simulink model "robusni_lin_regulacija_nelin_sim"  (R2020a)
settings: Solver=ode5  StartTime=0.0  StopTime=tfin  FixedStep=1e-4  RelTol=1e-3
values from neighbouring files (symbols this model uses):
  disturb_X = 0    [robusni_lin_regulacija_nelin_sim_matlab.m]
  F_lower_limit = 0    [robusni_lin_regulacija_nelin_sim_matlab.m]
  F_upper_limit = 1e-3*Fe    (= 0.00320891060125)    [robusni_lin_regulacija_nelin_sim_matlab.m]
  Fe = 3.20891060125344    (= 3.20891060125)    [robusni_lin_regulacija_nelin_sim_matlab.m]
  K1 = 0.03    [robusni_lin_regulacija_nelin_sim_matlab.m]
  K2 = 0.5    [robusni_lin_regulacija_nelin_sim_matlab.m]
  Kc1 = 1/abs(freqresp((1+1/Ti1/s)*G_design,w1_design))    [robusni_lin_regulacija_nelin_sim_matlab.m]
  mi_max = 1    [robusni_lin_regulacija_nelin_sim_matlab.m]
  S_step1 = delta    (= 0.0138373075366)    [robusni_lin_regulacija_nelin_sim_matlab.m]
  S_step2 = delta    (= 0.0138373075366)    [robusni_lin_regulacija_nelin_sim_matlab.m]
  S_time_step1 = 20    [robusni_lin_regulacija_nelin_sim_matlab.m]
  S_time_step2 = 50    [robusni_lin_regulacija_nelin_sim_matlab.m]
  Se = 0.218662692463450    (= 0.218662692463)    [robusni_lin_regulacija_nelin_sim_matlab.m]
  SF = 10    [robusni_lin_regulacija_nelin_sim_matlab.m]
  std_noise = 0    [robusni_lin_regulacija_nelin_sim_matlab.m]
  V = 4    [robusni_lin_regulacija_nelin_sim_matlab.m]
  x10 = Xe    (= 4.89066865377)    [robusni_lin_regulacija_nelin_sim_matlab.m]
  x20 = Se    (= 0.218662692463)    [robusni_lin_regulacija_nelin_sim_matlab.m]
  Y = Ynom    (= 0.5)    [robusni_lin_regulacija_nelin_sim_matlab.m]
  Y1 = Y - 0.2*Y    (= 0.4)    [robusni_lin_regulacija_nelin_sim_matlab.m]
  Y2 = Y - 0.1*Y    (= 0.45)    [robusni_lin_regulacija_nelin_sim_matlab.m]
  Y3 = Y + 0.1*Y    (= 0.55)    [robusni_lin_regulacija_nelin_sim_matlab.m]
  Y4 = Y + 0.2*Y    (= 0.6)    [robusni_lin_regulacija_nelin_sim_matlab.m]
undefined symbols (not defined in the file or in its folder): magnitude
libraries: cstblocks x10
settings Model: Creator=anaMceranic  LastModifiedBy=anaMceranic
settings DataIOCC: ReturnWorkspaceOutputs=off

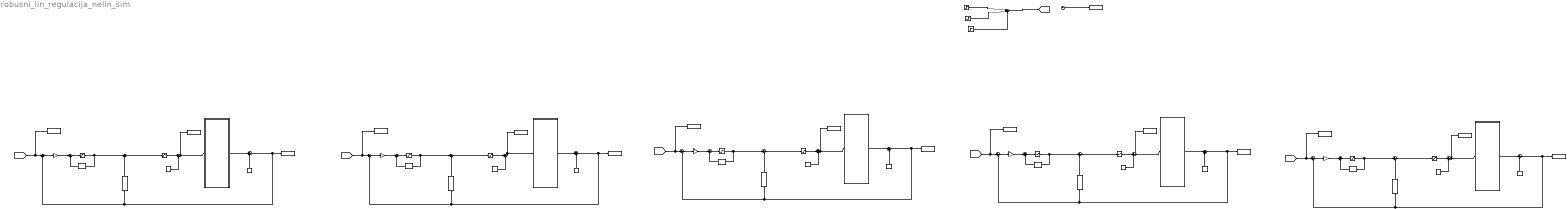
== system robusni_lin_regulacija_nelin_sim ==
  note: 1.2 Y
  note: 1.1 Y
  note: 0.9Y
  note: 0.8Y
  note: nominalni
  Clock : Clock
  Constant{1..5} (5 alike) : Constant  Value=Fe
  Gain{,1..4} (5 alike) : Gain  Gain=Kc1
  LTI System{,2,4,6,8} (5 alike) : cstblocks/LTI System  sys=KPI_aw  IC=[]
  LTI System{1,3,5,7,9} (5 alike) : cstblocks/LTI System  sys=Kfb  IC=[]
  Random Number{,1..4} (5 alike) : RandomNumber  Variance=std_noise  SampleTime=0.1
  Saturation{1..10} (10 alike) : Saturate  UpperLimit=F_upper_limit  LowerLimit=F_lower_limit
  Step2 : Step  Time=0  Before=Se  After=Se  SampleTime=0
  Step3 : Step  Time=S_time_step1  After=S_step1  SampleTime=0
  Step4 : Step  Time=S_time_step2  After=-S_step2  SampleTime=0
  Subsystem1 : Subsystem
  Subsystem2 : Subsystem
  Subsystem3 : Subsystem
  Subsystem4 : Subsystem
  Subsystem5 : Subsystem
  Sum{1..2,4,6,8,11..13,16..18,21..23,26} (15 alike) : Sum  Inputs=|++
  Sum{3,5,9..10,14..15,19..20,24..25} (10 alike) : Sum  Inputs=|+-
  Sum7 : Sum  Inputs=|+++
  To Workspace1 : ToWorkspace  VariableName=t_out  SampleTime=-1
  To Workspace10 : ToWorkspace  VariableName=S_ref_out2  SampleTime=-1
  To Workspace11 : ToWorkspace  VariableName=S_out3  SampleTime=-1
  To Workspace12 : ToWorkspace  VariableName=F_out3  SampleTime=-1
  To Workspace13 : ToWorkspace  VariableName=S_ref_out3  SampleTime=-1
  To Workspace14 : ToWorkspace  VariableName=S_out4  SampleTime=-1
  To Workspace15 : ToWorkspace  VariableName=F_out4  SampleTime=-1
  To Workspace16 : ToWorkspace  VariableName=S_ref_out4  SampleTime=-1
  To Workspace2 : ToWorkspace  VariableName=S_out1  SampleTime=-1
  To Workspace3 : ToWorkspace  VariableName=F_out1  SampleTime=-1
  To Workspace4 : ToWorkspace  VariableName=S_ref_out1  SampleTime=-1
  To Workspace5 : ToWorkspace  VariableName=S_out2  SampleTime=-1
  To Workspace6 : ToWorkspace  VariableName=S_out  SampleTime=-1
  To Workspace7 : ToWorkspace  VariableName=F_out  SampleTime=-1
  To Workspace8 : ToWorkspace  VariableName=S_ref_out  SampleTime=-1
  To Workspace9 : ToWorkspace  VariableName=F_out2  SampleTime=-1
  wires:
  Clock/1 -> To Workspace1/1
  Sum6/1 -> To Workspace7/1, Subsystem2/1(u)
  Saturation1/1 -> Sum6/1
  Constant1/1 -> Sum6/2
  Sum5/1 -> Gain/1
  Sum7/1 -> [S_refere]
  Step2/1 -> Sum7/1
  [S_refere] -> To Workspace8/1, Sum5/1
  Gain/1 -> Sum1/1
  Sum1/1 -> Saturation2/1
  LTI System/1 -> Sum1/2
  Step3/1 -> Sum7/2
  Step4/1 -> Sum7/3
  Subsystem2/1(y) -> Sum2/1
  Sum2/1 -> Sum5/2, LTI System1/1, To Workspace6/1
  Random Number/1 -> Sum2/2
  Saturation2/1 -> Sum3/1, LTI System/1
  Sum3/1 -> Saturation1/1
  LTI System1/1 -> Sum3/2
  Sum4/1 -> Saturation4/1
  Constant2/1 -> Sum11/2
  Sum11/1 -> To Workspace3/1, Subsystem1/1(u)
  Gain1/1 -> Sum4/1
  Sum9/1 -> Saturation3/1
  Saturation4/1 -> Sum9/1, LTI System2/1
  LTI System2/1 -> Sum4/2
  Saturation3/1 -> Sum11/1
  Sum8/1 -> Sum10/2, LTI System3/1, To Workspace2/1
  Random Number1/1 -> Sum8/2
  [S_refere] -> To Workspace4/1, Sum10/1
  LTI System3/1 -> Sum9/2
  Subsystem1/1(y) -> Sum8/1
  Sum10/1 -> Gain1/1
  Sum12/1 -> Saturation6/1
  Constant3/1 -> Sum16/2
  Sum16/1 -> To Workspace9/1, Subsystem3/1(u)
  Gain2/1 -> Sum12/1
  Sum14/1 -> Saturation5/1
  Saturation6/1 -> Sum14/1, LTI System4/1
  LTI System4/1 -> Sum12/2
  Saturation5/1 -> Sum16/1
  Sum13/1 -> Sum15/2, LTI System5/1, To Workspace5/1
  Random Number2/1 -> Sum13/2
  [S_refere] -> To Workspace10/1, Sum15/1
  LTI System5/1 -> Sum14/2
  Subsystem3/1(y) -> Sum13/1
  Sum15/1 -> Gain2/1
  Sum17/1 -> Saturation8/1
  Constant4/1 -> Sum21/2
  Sum21/1 -> To Workspace12/1, Subsystem4/1(u)
  Gain3/1 -> Sum17/1
  Sum19/1 -> Saturation7/1
  Saturation8/1 -> Sum19/1, LTI System6/1
  LTI System6/1 -> Sum17/2
  Saturation7/1 -> Sum21/1
  Sum18/1 -> Sum20/2, LTI System7/1, To Workspace11/1
  Random Number3/1 -> Sum18/2
  [S_refere] -> To Workspace13/1, Sum20/1
  LTI System7/1 -> Sum19/2
  Subsystem4/1(y) -> Sum18/1
  Sum20/1 -> Gain3/1
  Sum22/1 -> Saturation10/1
  Constant5/1 -> Sum26/2
  Sum26/1 -> To Workspace15/1, Subsystem5/1(u)
  Gain4/1 -> Sum22/1
  Sum24/1 -> Saturation9/1
  Saturation10/1 -> Sum24/1, LTI System8/1
  LTI System8/1 -> Sum22/2
  Saturation9/1 -> Sum26/1
  Sum23/1 -> Sum25/2, LTI System9/1, To Workspace14/1
  Random Number4/1 -> Sum23/2
  [S_refere] -> To Workspace16/1, Sum25/1
  LTI System9/1 -> Sum24/2
  Subsystem5/1(y) -> Sum23/1
  Sum25/1 -> Gain4/1

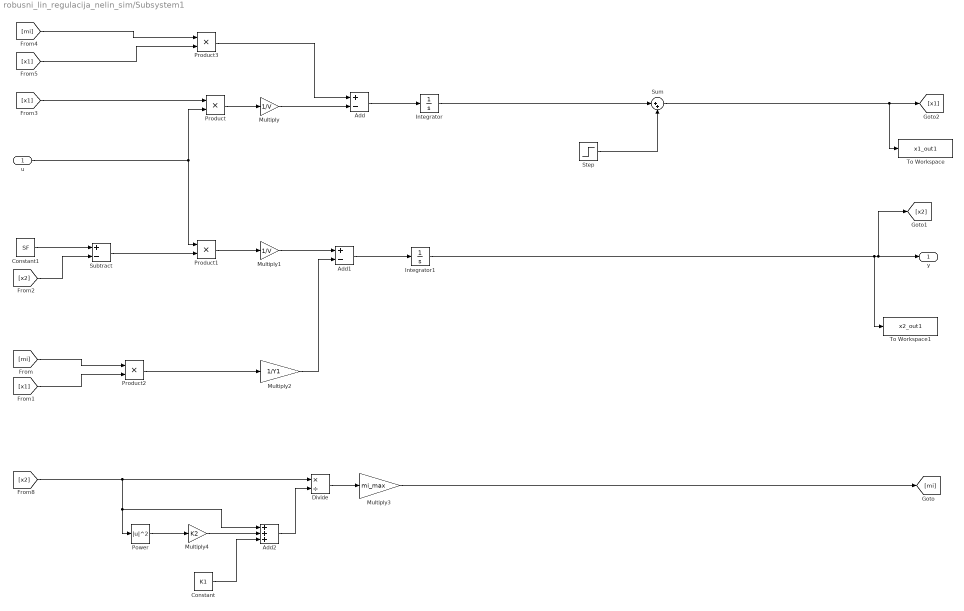
== system robusni_lin_regulacija_nelin_sim/Subsystem1 ==
  u : Inport
  Add : Sum  Inputs=+-
  Add1 : Sum  Inputs=+-
  Add2 : Sum  Inputs=+++
  Constant : Constant  Value=K1
  Constant1 : Constant  Value=SF
  Divide : Product  Inputs=*/
  Integrator : Integrator  InitialCondition=x10
  Integrator1 : Integrator  InitialCondition=x20
  Multiply : Gain  Gain=1/V
  Multiply1 : Gain  Gain=1/V
  Multiply2 : Gain  Gain=1/Y1
  Multiply3 : Gain  Gain=mi_max
  Multiply4 : Gain  Gain=K2
  Power : Math  Operator=magnitude^2  SaturateOnIntegerOverflow=on
  Product{,1..3} (4 alike) : Product
  Step : Step  Time=2  After=disturb_X  SampleTime=0
  Subtract : Sum  Inputs=+-
  Sum : Sum  Inputs=|++
  To Workspace : ToWorkspace  VariableName=x1_out1  SampleTime=-1
  To Workspace1 : ToWorkspace  VariableName=x2_out1  SampleTime=-1
  y : Outport
  wires:
  [x1] -> Product2/2
  Product2/1 -> Multiply2/1
  Multiply/1 -> Add/2
  Add2/1 -> Divide/2
  Constant/1 -> Add2/3
  [x1] -> Product3/2
  Multiply4/1 -> Add2/2
  [mi] -> Product2/1
  Multiply3/1 -> [mi]
  Power/1 -> Multiply4/1
  Constant1/1 -> Subtract/1
  [x2] -> Subtract/2
  Add1/1 -> Integrator1/1
  Multiply2/1 -> Add1/2
  Integrator1/1 -> [x2], y/1, To Workspace1/1
  Divide/1 -> Multiply3/1
  Product3/1 -> Add/1
  u/1 -> Product1/1, Product/2
  [x1] -> Product/1
  Multiply1/1 -> Add1/1
  Product1/1 -> Multiply1/1
  Subtract/1 -> Product1/2
  [x2] -> Divide/1, Add2/1, Power/1
  Add/1 -> Integrator/1
  Product/1 -> Multiply/1
  [mi] -> Product3/1
  Integrator/1 -> Sum/1
  Sum/1 -> To Workspace/1, [x1]
  Step/1 -> Sum/2

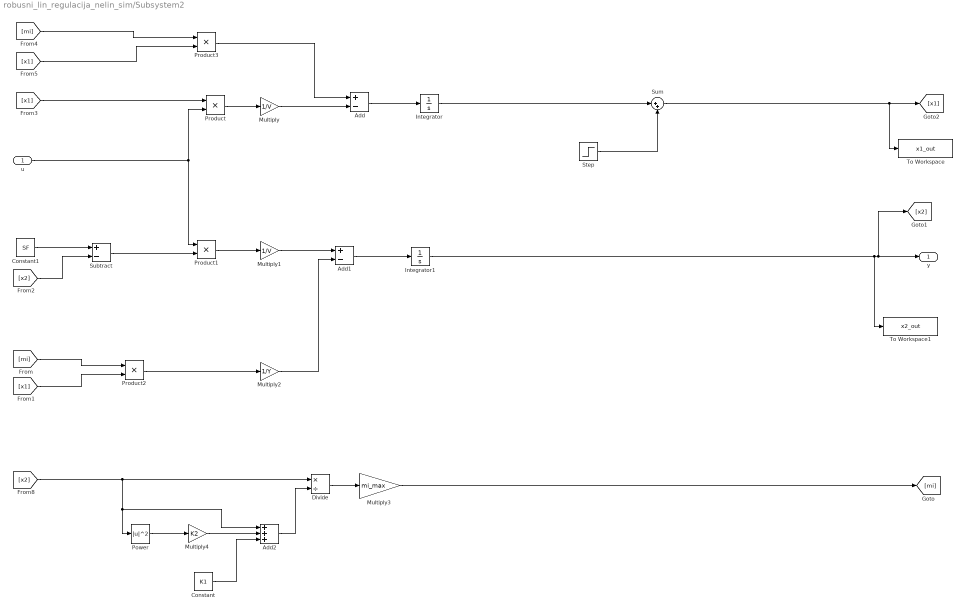
== system robusni_lin_regulacija_nelin_sim/Subsystem2 ==
  u : Inport
  Add : Sum  Inputs=+-
  Add1 : Sum  Inputs=+-
  Add2 : Sum  Inputs=+++
  Constant : Constant  Value=K1
  Constant1 : Constant  Value=SF
  Divide : Product  Inputs=*/
  Integrator : Integrator  InitialCondition=x10
  Integrator1 : Integrator  InitialCondition=x20
  Multiply : Gain  Gain=1/V
  Multiply1 : Gain  Gain=1/V
  Multiply2 : Gain  Gain=1/Y
  Multiply3 : Gain  Gain=mi_max
  Multiply4 : Gain  Gain=K2
  Power : Math  Operator=magnitude^2  SaturateOnIntegerOverflow=on
  Product{,1..3} (4 alike) : Product
  Step : Step  Time=2  After=disturb_X  SampleTime=0
  Subtract : Sum  Inputs=+-
  Sum : Sum  Inputs=|++
  To Workspace : ToWorkspace  VariableName=x1_out  SampleTime=-1
  To Workspace1 : ToWorkspace  VariableName=x2_out  SampleTime=-1
  y : Outport
  wires:
  [x1] -> Product2/2
  Product2/1 -> Multiply2/1
  Multiply/1 -> Add/2
  Add2/1 -> Divide/2
  Constant/1 -> Add2/3
  [x1] -> Product3/2
  Multiply4/1 -> Add2/2
  [mi] -> Product2/1
  Multiply3/1 -> [mi]
  Power/1 -> Multiply4/1
  Constant1/1 -> Subtract/1
  [x2] -> Subtract/2
  Add1/1 -> Integrator1/1
  Multiply2/1 -> Add1/2
  Integrator1/1 -> [x2], y/1, To Workspace1/1
  Divide/1 -> Multiply3/1
  Product3/1 -> Add/1
  u/1 -> Product1/1, Product/2
  [x1] -> Product/1
  Multiply1/1 -> Add1/1
  Product1/1 -> Multiply1/1
  Subtract/1 -> Product1/2
  [x2] -> Divide/1, Add2/1, Power/1
  Add/1 -> Integrator/1
  Product/1 -> Multiply/1
  [mi] -> Product3/1
  Integrator/1 -> Sum/1
  Sum/1 -> To Workspace/1, [x1]
  Step/1 -> Sum/2

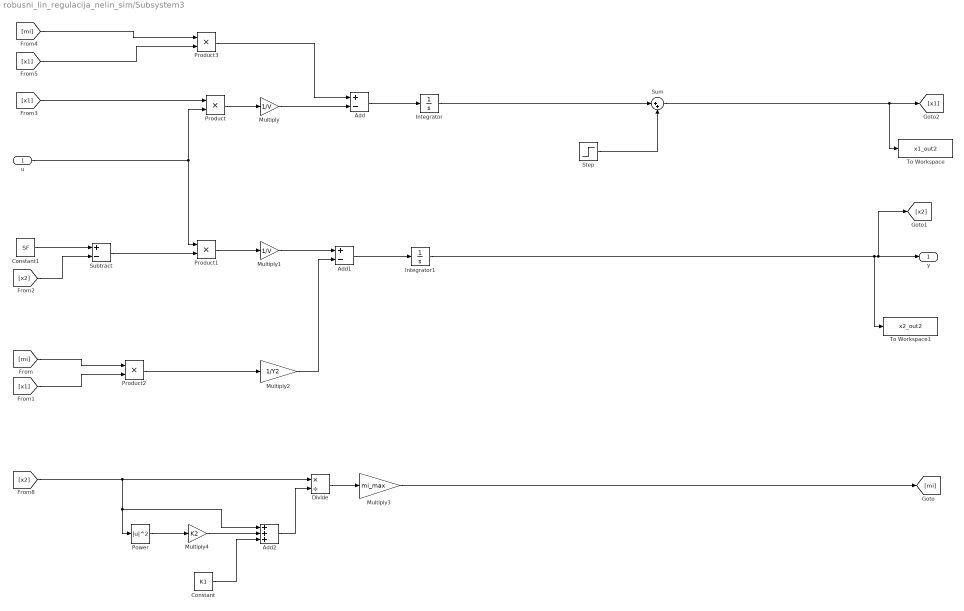
== system robusni_lin_regulacija_nelin_sim/Subsystem3 ==
  u : Inport
  Add : Sum  Inputs=+-
  Add1 : Sum  Inputs=+-
  Add2 : Sum  Inputs=+++
  Constant : Constant  Value=K1
  Constant1 : Constant  Value=SF
  Divide : Product  Inputs=*/
  Integrator : Integrator  InitialCondition=x10
  Integrator1 : Integrator  InitialCondition=x20
  Multiply : Gain  Gain=1/V
  Multiply1 : Gain  Gain=1/V
  Multiply2 : Gain  Gain=1/Y2
  Multiply3 : Gain  Gain=mi_max
  Multiply4 : Gain  Gain=K2
  Power : Math  Operator=magnitude^2  SaturateOnIntegerOverflow=on
  Product{,1..3} (4 alike) : Product
  Step : Step  Time=2  After=disturb_X  SampleTime=0
  Subtract : Sum  Inputs=+-
  Sum : Sum  Inputs=|++
  To Workspace : ToWorkspace  VariableName=x1_out2  SampleTime=-1
  To Workspace1 : ToWorkspace  VariableName=x2_out2  SampleTime=-1
  y : Outport
  wires:
  [x1] -> Product2/2
  Product2/1 -> Multiply2/1
  Multiply/1 -> Add/2
  Add2/1 -> Divide/2
  Constant/1 -> Add2/3
  [x1] -> Product3/2
  Multiply4/1 -> Add2/2
  [mi] -> Product2/1
  Multiply3/1 -> [mi]
  Power/1 -> Multiply4/1
  Constant1/1 -> Subtract/1
  [x2] -> Subtract/2
  Add1/1 -> Integrator1/1
  Multiply2/1 -> Add1/2
  Integrator1/1 -> [x2], y/1, To Workspace1/1
  Divide/1 -> Multiply3/1
  Product3/1 -> Add/1
  u/1 -> Product1/1, Product/2
  [x1] -> Product/1
  Multiply1/1 -> Add1/1
  Product1/1 -> Multiply1/1
  Subtract/1 -> Product1/2
  [x2] -> Divide/1, Add2/1, Power/1
  Add/1 -> Integrator/1
  Product/1 -> Multiply/1
  [mi] -> Product3/1
  Integrator/1 -> Sum/1
  Sum/1 -> To Workspace/1, [x1]
  Step/1 -> Sum/2

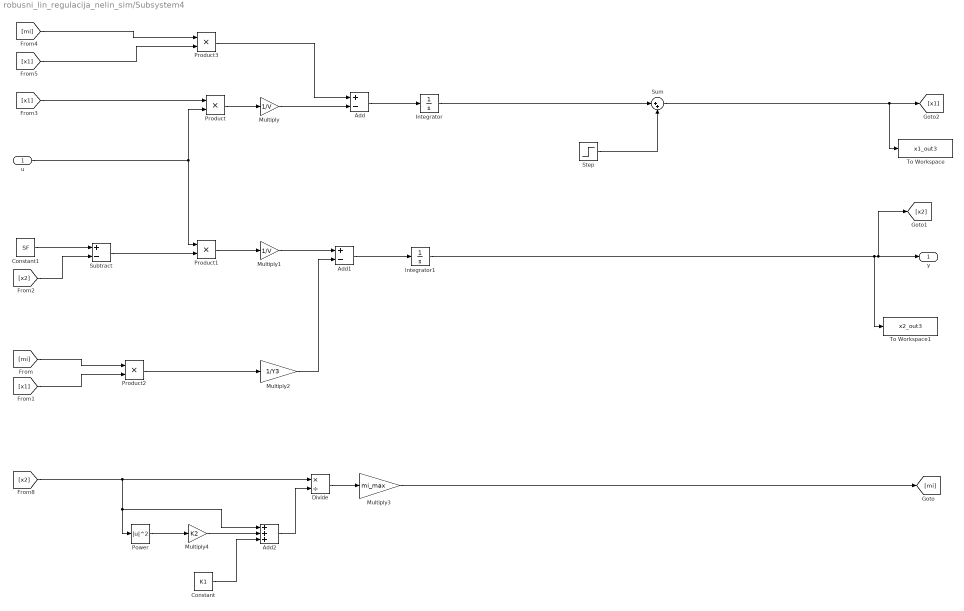
== system robusni_lin_regulacija_nelin_sim/Subsystem4 ==
  u : Inport
  Add : Sum  Inputs=+-
  Add1 : Sum  Inputs=+-
  Add2 : Sum  Inputs=+++
  Constant : Constant  Value=K1
  Constant1 : Constant  Value=SF
  Divide : Product  Inputs=*/
  Integrator : Integrator  InitialCondition=x10
  Integrator1 : Integrator  InitialCondition=x20
  Multiply : Gain  Gain=1/V
  Multiply1 : Gain  Gain=1/V
  Multiply2 : Gain  Gain=1/Y3
  Multiply3 : Gain  Gain=mi_max
  Multiply4 : Gain  Gain=K2
  Power : Math  Operator=magnitude^2  SaturateOnIntegerOverflow=on
  Product{,1..3} (4 alike) : Product
  Step : Step  Time=2  After=disturb_X  SampleTime=0
  Subtract : Sum  Inputs=+-
  Sum : Sum  Inputs=|++
  To Workspace : ToWorkspace  VariableName=x1_out3  SampleTime=-1
  To Workspace1 : ToWorkspace  VariableName=x2_out3  SampleTime=-1
  y : Outport
  wires:
  [x1] -> Product2/2
  Product2/1 -> Multiply2/1
  Multiply/1 -> Add/2
  Add2/1 -> Divide/2
  Constant/1 -> Add2/3
  [x1] -> Product3/2
  Multiply4/1 -> Add2/2
  [mi] -> Product2/1
  Multiply3/1 -> [mi]
  Power/1 -> Multiply4/1
  Constant1/1 -> Subtract/1
  [x2] -> Subtract/2
  Add1/1 -> Integrator1/1
  Multiply2/1 -> Add1/2
  Integrator1/1 -> [x2], y/1, To Workspace1/1
  Divide/1 -> Multiply3/1
  Product3/1 -> Add/1
  u/1 -> Product1/1, Product/2
  [x1] -> Product/1
  Multiply1/1 -> Add1/1
  Product1/1 -> Multiply1/1
  Subtract/1 -> Product1/2
  [x2] -> Divide/1, Add2/1, Power/1
  Add/1 -> Integrator/1
  Product/1 -> Multiply/1
  [mi] -> Product3/1
  Integrator/1 -> Sum/1
  Sum/1 -> To Workspace/1, [x1]
  Step/1 -> Sum/2

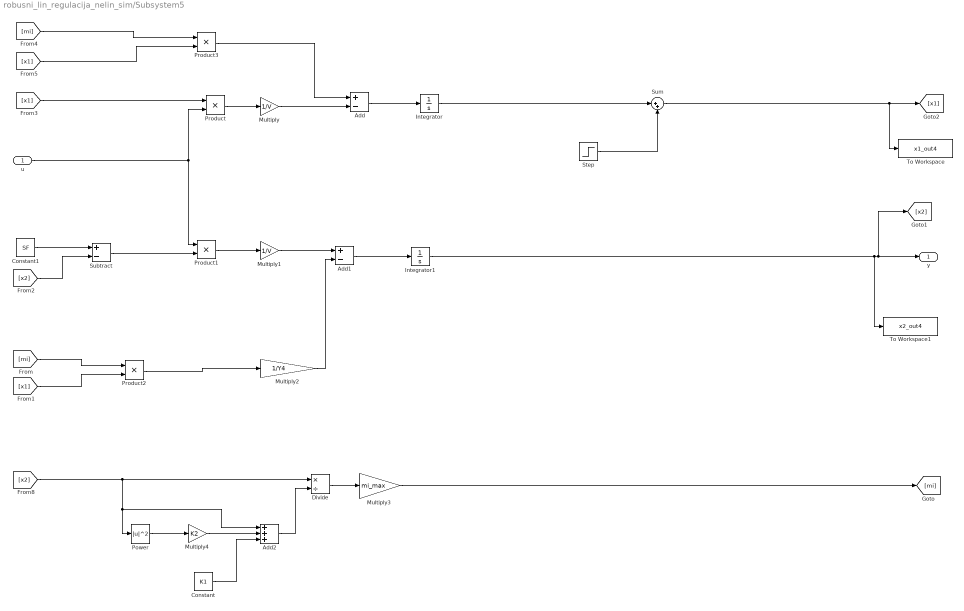
== system robusni_lin_regulacija_nelin_sim/Subsystem5 ==
  u : Inport
  Add : Sum  Inputs=+-
  Add1 : Sum  Inputs=+-
  Add2 : Sum  Inputs=+++
  Constant : Constant  Value=K1
  Constant1 : Constant  Value=SF
  Divide : Product  Inputs=*/
  Integrator : Integrator  InitialCondition=x10
  Integrator1 : Integrator  InitialCondition=x20
  Multiply : Gain  Gain=1/V
  Multiply1 : Gain  Gain=1/V
  Multiply2 : Gain  Gain=1/Y4
  Multiply3 : Gain  Gain=mi_max
  Multiply4 : Gain  Gain=K2
  Power : Math  Operator=magnitude^2  SaturateOnIntegerOverflow=on
  Product{,1..3} (4 alike) : Product
  Step : Step  Time=2  After=disturb_X  SampleTime=0
  Subtract : Sum  Inputs=+-
  Sum : Sum  Inputs=|++
  To Workspace : ToWorkspace  VariableName=x1_out4  SampleTime=-1
  To Workspace1 : ToWorkspace  VariableName=x2_out4  SampleTime=-1
  y : Outport
  wires:
  [x1] -> Product2/2
  Product2/1 -> Multiply2/1
  Multiply/1 -> Add/2
  Add2/1 -> Divide/2
  Constant/1 -> Add2/3
  [x1] -> Product3/2
  Multiply4/1 -> Add2/2
  [mi] -> Product2/1
  Multiply3/1 -> [mi]
  Power/1 -> Multiply4/1
  Constant1/1 -> Subtract/1
  [x2] -> Subtract/2
  Add1/1 -> Integrator1/1
  Multiply2/1 -> Add1/2
  Integrator1/1 -> [x2], y/1, To Workspace1/1
  Divide/1 -> Multiply3/1
  Product3/1 -> Add/1
  u/1 -> Product1/1, Product/2
  [x1] -> Product/1
  Multiply1/1 -> Add1/1
  Product1/1 -> Multiply1/1
  Subtract/1 -> Product1/2
  [x2] -> Divide/1, Add2/1, Power/1
  Add/1 -> Integrator/1
  Product/1 -> Multiply/1
  [mi] -> Product3/1
  Integrator/1 -> Sum/1
  Sum/1 -> To Workspace/1, [x1]
  Step/1 -> Sum/2
